simulink model "Houghline_real_nocolor_2"  (R2016a)
settings: Solver=VariableStepAuto  StartTime=0.0  StopTime=inf  RelTol=1e-3
undefined symbols (not defined in the file): gray, Rec, SDTV
libraries: visionconversions x4, visiontransforms x3, visionfilter x2, visiontextngfix x2, dspvision x1, visionanalysis x1, visionstatistics x1
settings Model: Creator=Yewly  LastModifiedBy=Yewly
settings GRTTargetCC: GeneratePreprocessorConditionals=Use local settings

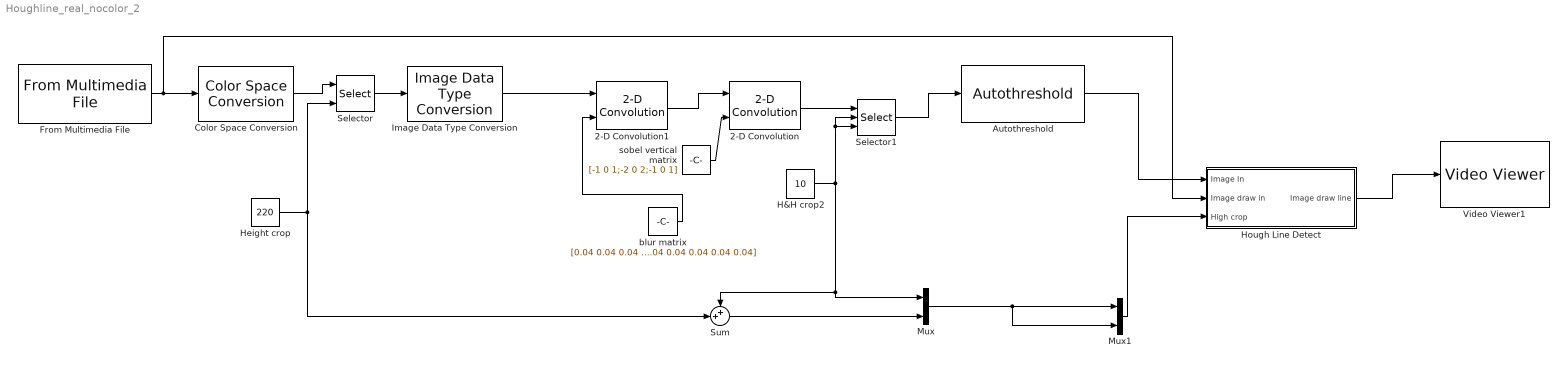
== system Houghline_real_nocolor_2 ==
  2-D Convolution : visionfilter/2-D Convolution  outSize=Full  normalize=off  outputMode=Binary point scaling  outputWordLength=32  outputFracLength=12  prodOutputMode=Binary point scaling  prodOutputWordLength=32  prodOutputFracLength=10  roundingMode=Floor  overflowMode=off
  2-D Convolution1 : visionfilter/2-D Convolution  outSize=Full  normalize=off  outputMode=Binary point scaling  outputWordLength=32  outputFracLength=12  prodOutputMode=Binary point scaling  prodOutputWordLength=32  prodOutputFracLength=10  roundingMode=Floor  overflowMode=off
  Autothreshold : visionconversions/Autothreshold  operator=>  threshOut=off  effMetricOut=off  userDefinedRange=off  umin=0  umax=255  outOfRngOpt=Warn and saturate  scaleThreshold=off  scaleFactor=1  P1Mode=Specify word length  P1WordLength=32  P1FracLength=30  P2Mode=Specify word length  P2WordLength=32  P2FracLength=22  P3Mode=Specify word length  P3WordLength=32  P3FracLength=14  P4Mode=Binary point scaling  P4WordLength=32  P4FracLength=15  Q1Mode=Specify word length  Q1WordLength=32  Q1FracLength=16  EMMode=Specify word length  EMWordLength=16  EMFracLength=14  roundingMode=Floor  overflowMode=off
  Color Space Conversion : visionconversions/Color Space  Conversion  conversion=Obsolete  conversionActive=R'G'B' to intensity  wp_str=D65  rec=Rec. 601 (SDTV)  sys=1125/60/2:1  imagePorts=One multidimensional signal
  From Multimedia File : dspvision/From Multimedia File  inputFilename=lane3.mp4  loop=on  numPlays=inf  outputStreams=Video only  videoDataType=single  audioDataType=int16  inheritSampleTime=on  userDefinedSampleTime=1/5  noAudioOutput=off  isIntensityVideo=off  fourcc=RGB  colorVideoFormat=One multidimensional signal  outputEOF=off  dataOrg=Column-major  audioFrameSize=1024  computeAudioFrameSize=off  outSamplingMode=Sample based
  H&H crop2 : Constant  Value=10  OutDataTypeStr=double
  Height crop : Constant  Value=220  OutDataTypeStr=double
  "Hough Line Detect " : Subsystem
  Image Data Type Conversion : visionconversions/Image Data Type Conversion  outDT=double  isSigned=on  wordLen=16  numFracBits=0
  Mux : Mux  Inputs=2
  Mux1 : Mux  Inputs=2
  Selector : Selector  NumberOfDimensions=2  InputPortWidth=3  IndexOptions=Starting index (port),Select all  Indices=220,1  OutputSizes=220,1
  Selector1 : Selector  NumberOfDimensions=2  InputPortWidth=3  IndexOptions=Starting index (port),Starting index (port)  Indices=10,10  OutputSizes=210,630
  Sum : Sum  Inputs=++|
  Video Viewer1 : VideoViewer  colormapValue=gray(256)  FigPos=[7.4 550 526.4 444.8]
  blur matrix : Constant  Value=[0.04 0.04 0.04 0.04 0.04;0.04 0.04 0.04 0.04 0.04;0.04 0.04 0.04 0.04 0.04;0.04 0.04 0.04 0.04 0.04;0.04 0.04 0.04 0.04 0.04]  OutDataTypeStr=double
  sobel vertical matrix : Constant  Value=[-1 0 1;-2 0 2;-1 0 1]  OutDataTypeStr=double
  wires:
  "Hough Line Detect "/1("Image draw line ") -> Video Viewer1/1
  From Multimedia File/1 -> "Hough Line Detect "/2("Image draw in "), Color Space Conversion/1
  Color Space Conversion/1 -> Selector/1
  Autothreshold/1 -> "Hough Line Detect "/1(Image In)
  Selector/1 -> Image Data Type Conversion/1
  2-D Convolution/1 -> Selector1/1
  2-D Convolution1/1 -> 2-D Convolution/1
  Selector1/1 -> Autothreshold/1
  Image Data Type Conversion/1 -> 2-D Convolution1/1
  blur matrix/1 -> 2-D Convolution1/2
  sobel vertical matrix/1 -> 2-D Convolution/2
  Height crop/1 -> Sum/2, Selector/2
  Mux/1 -> Mux1/2, Mux1/1
  Mux1/1 -> "Hough Line Detect "/3(High crop)
  H&H crop2/1 -> Selector1/3, Selector1/2, Mux/1, Sum/1
  Sum/1 -> Mux/2

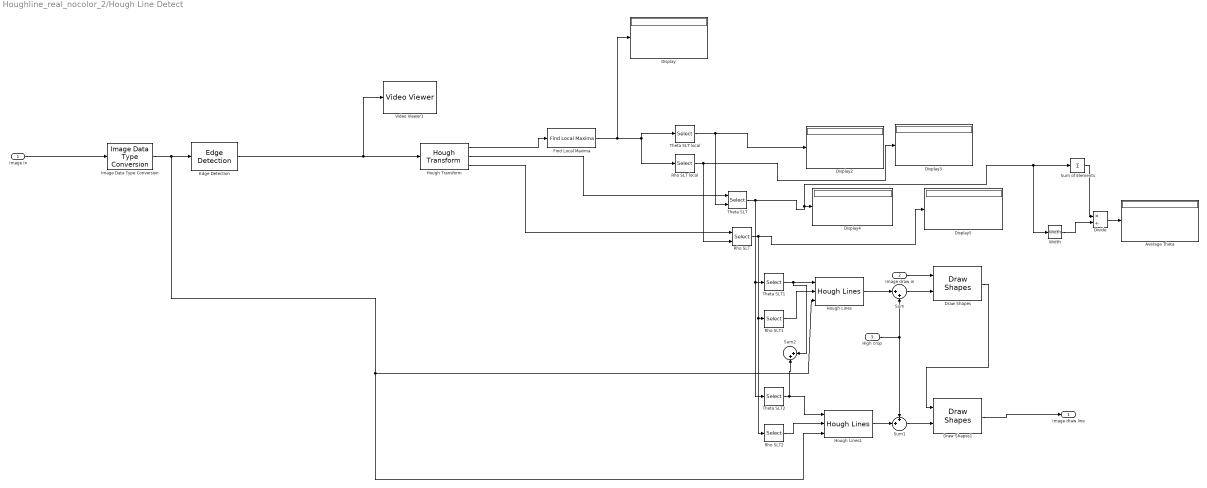
== system Houghline_real_nocolor_2/Hough Line Detect  ==
  Image In : Inport
  "Image draw in " : Inport  Port=2
  High crop : Inport  Port=3
  Average Theta : Display
  Display{,2..5} (5 alike) : Display
  Divide : Product  Inputs=*/
  Draw Shapes : visiontextngfix/Draw Shapes  shape=Lines  fill=off  lineWidth=10  fillClrSource=Specify via dialog  display=User-specified value  intensity=200  color=[255 0 0]  opacity=0.6  viewport=Entire image  antialiasing=off  inType=Obsolete  imagePorts=One multidimensional signal  prodOutputMode=Binary point scaling  prodOutputWordLength=32  prodOutputFracLength=14  memoryMode=Specify word length  memoryWordLength=16  memoryFracLength=14  roundingMode=Floor  overflowMode=off
  Draw Shapes1 : visiontextngfix/Draw Shapes  shape=Lines  fill=off  lineWidth=10  fillClrSource=Specify via dialog  display=User-specified value  intensity=200  color=[0 0 255]  opacity=0.6  viewport=Entire image  antialiasing=off  inType=Obsolete  imagePorts=One multidimensional signal  prodOutputMode=Binary point scaling  prodOutputWordLength=32  prodOutputFracLength=14  memoryMode=Specify word length  memoryWordLength=16  memoryFracLength=14  roundingMode=Floor  overflowMode=off
  Edge Detection : visionanalysis/Edge Detection  method=Sobel  outputType=Binary image  userDefinedThreshold=off  thresholdSource=Specify via dialog  threshold=20  thresholdTuning=4  edgeThinning=on  threshold_canny=[0.25 0.60]  autoPercent=70  sigma=1  prodOutputMode=Binary point scaling  prodOutputWordLength=32  prodOutputFracLength=8  roundingMode=Floor  overflowMode=off
  Find Local Maxima : visionstatistics/Find Local Maxima  num_peaks=100  nhood_size=[5 7]  src_thresh=Obsolete9b  src_thresh_inuse=Specify via dialog  threshold=10  inputIsHough=on  dt_peak=uint32  isOutVarDim=on  dt_count=uint32
  Hough Lines : visiontransforms/Hough Lines  sineCompMethod=Trigonometric function  thetaRes=pi/180  firstCoeffMode=Specify word length  firstCoeffWordLength=16  firstCoeffFracLength=15  prodOutputMode=Binary point scaling  prodOutputWordLength=32  prodOutputFracLength=16  roundingMode=Nearest  overflowMode=on
  Hough Lines1 : visiontransforms/Hough Lines  sineCompMethod=Trigonometric function  thetaRes=pi/180  firstCoeffMode=Specify word length  firstCoeffWordLength=16  firstCoeffFracLength=15  prodOutputMode=Binary point scaling  prodOutputWordLength=32  prodOutputFracLength=16  roundingMode=Nearest  overflowMode=on
  Hough Transform : visiontransforms/Hough Transform  theta_res=pi/360  rho_res=1  out_theta_rho=on  outdtmode=double  firstCoeffMode=Binary point scaling  firstCoeffWordLength=16  firstCoeffFracLength=14  secondCoeffMode=Binary point scaling  secondCoeffWordLength=32  secondCoeffFracLength=16  outputMode=Binary point scaling  outputWordLength=16  outputFracLength=0  accumMode=Binary point scaling  accumWordLength=32  accumFracLength=20  prodOutputMode=Binary point scaling  prodOutputWordLength=32  prodOutputFracLength=20  memoryMode=Binary point scaling  memoryWordLength=32  memoryFracLength=16  roundingMode=Nearest  overflowMode=on
  Image Data Type Conversion : visionconversions/Image Data Type Conversion  outDT=double  isSigned=on  wordLen=16  numFracBits=0
  Rho SLT : Selector  NumberOfDimensions=2  InputPortWidth=3  IndexOptions=Index vector (dialog),Index vector (port)  Indices=1,1  OutputSizes=1,1
  Rho SLT local : Selector  NumberOfDimensions=2  InputPortWidth=2  IndexOptions=Starting index (dialog),Index vector (dialog)  Indices=1,2  OutputSizes=60,1
  Rho SLT1 : Selector  NumberOfDimensions=2  InputPortWidth=3  IndexOptions=Index vector (dialog),Index vector (dialog)  Indices=1,1  OutputSizes=1,1
  Rho SLT2 : Selector  NumberOfDimensions=2  InputPortWidth=3  IndexOptions=Index vector (dialog),Index vector (dialog)  Indices=1,3  OutputSizes=1,1
  Sum : Sum  Inputs=|++
  Sum of Elements : Sum  Inputs=+
  Sum1 : Sum  Inputs=++|
  Sum2 : Sum  Inputs=|++
  Theta SLT : Selector  NumberOfDimensions=2  InputPortWidth=3  IndexOptions=Index vector (dialog),Index vector (port)  Indices=1,1  OutputSizes=1,1
  Theta SLT local : Selector  NumberOfDimensions=2  InputPortWidth=2  IndexOptions=Starting index (dialog),Index vector (dialog)  Indices=1,1  OutputSizes=60,1
  Theta SLT1 : Selector  NumberOfDimensions=2  InputPortWidth=3  IndexOptions=Index vector (dialog),Index vector (dialog)  Indices=1,1  OutputSizes=1,1
  Theta SLT2 : Selector  NumberOfDimensions=2  InputPortWidth=3  IndexOptions=Index vector (dialog),Index vector (dialog)  Indices=1,3  OutputSizes=1,1
  Video Viewer1 : VideoViewer  colormapValue=gray(256)  FigPos=[9.8 810.8 563.2 205.6]
  Width : Width
  "Image draw line " : Outport
  wires:
  Draw Shapes1/1 -> "Image draw line "/1
  Hough Transform/1 -> Find Local Maxima/1
  Draw Shapes/1 -> Draw Shapes1/1
  Image Data Type Conversion/1 -> Hough Lines1/3, Hough Lines/3, Edge Detection/1
  Find Local Maxima/1 -> Display/1, Rho SLT local/1, Theta SLT local/1
  Image In/1 -> Image Data Type Conversion/1
  "Image draw in "/1 -> Draw Shapes/1
  Edge Detection/1 -> Video Viewer1/1, Hough Transform/1
  Hough Transform/2 -> Theta SLT/1
  Hough Transform/3 -> Rho SLT/1
  Theta SLT local/1 -> Theta SLT/2, Display2/1
  Rho SLT local/1 -> Rho SLT/2, Display3/1
  Rho SLT/1 -> Rho SLT2/1, Rho SLT1/1, Display5/1
  Theta SLT/1 -> Theta SLT2/1, Theta SLT1/1, Width/1, Sum of Elements/1, Display4/1
  Sum of Elements/1 -> Divide/1
  Theta SLT1/1 -> Sum2/1, Hough Lines/1
  Rho SLT1/1 -> Hough Lines/2
  Theta SLT2/1 -> Hough Lines1/1, Sum2/2
  Rho SLT2/1 -> Hough Lines1/2
  Hough Lines/1 -> Sum/1
  Sum/1 -> Draw Shapes/2
  High crop/1 -> Sum/2, Sum1/1
  Sum1/1 -> Draw Shapes1/2
  Hough Lines1/1 -> Sum1/2
  Width/1 -> Divide/2
  Divide/1 -> Average Theta/1
